simulink model "s_heli3d_cnn"  (R2023a)
settings: Solver=ode1  StartTime=0.0  StopTime=30  FixedStep=0.002  RelTol=1e-3  EnableMultiTasking=on
model workspace (MAT data in the model file):
  helicopter_models.Mdl = SeriesNetwork
  helicopter_models.Mdl.any.Version = 1
  helicopter_models.Mdl.any.Layers(1) = nnet.cnn.layer.FeatureInputLayer
  helicopter_models.Mdl.any.Layers(1).any.Version = 2
  helicopter_models.Mdl.any.Layers(1).any.Name = 'input'
  helicopter_models.Mdl.any.Layers(1).any.InputSize = 9
  helicopter_models.Mdl.any.Layers(1).any.Normalization = []
  helicopter_models.Mdl.any.Layers(1).any.NormalizationDimension = 'auto'
  helicopter_models.Mdl.any.Layers(1).any.SplitComplexInputs = 0
  helicopter_models.Mdl.any.Layers(2) = nnet.cnn.layer.FullyConnectedLayer
  helicopter_models.Mdl.any.Layers(2).any.Version = 3
  helicopter_models.Mdl.any.Layers(2).any.Name = 'fc1'
  helicopter_models.Mdl.any.Layers(2).any.InputSize = 9
  helicopter_models.Mdl.any.Layers(2).any.OutputSize = 256
  helicopter_models.Mdl.any.Layers(2).any.Weights.Version = 2
  helicopter_models.Mdl.any.Layers(2).any.Weights.Value = [0.13310675323 0.208178877831 -0.160442724824 0.136672541499 0.137998655438 0.0987144708633 0.0352399460971 -0.192555785179 0.245779588819 0.00993849057704 -0.0564966723323 -0.160766735673 ... (2304 elements, 256x9)]
  helicopter_models.Mdl.any.Layers(2).any.Weights.LearnRateFactor = 1
  helicopter_models.Mdl.any.Layers(2).any.Weights.L2Factor = 1
  helicopter_models.Mdl.any.Layers(2).any.Weights.Initializer.Version = 1
  helicopter_models.Mdl.any.Layers(2).any.Weights.Initializer.Class = 'nnet.internal.cnn.layer.learnable.initializer.Glorot'
  helicopter_models.Mdl.any.Layers(2).any.Weights.Initializer.ConstructorArguments = {2, 1}
  helicopter_models.Mdl.any.Layers(2).any.Bias.Version = 2
  helicopter_models.Mdl.any.Layers(2).any.Bias.Value = [0.149443045259 0.102787695825 0.0137507077307 -0.0149580715224 -0.377757281065 0.0530572384596 -0.0382270552218 0.0523963347077 0.0614480637014 -0.112386830151 -0.0184559673071 0.0208104513586 ... (256 elements, 256x1)]
  helicopter_models.Mdl.any.Layers(2).any.Bias.LearnRateFactor = 1
  helicopter_models.Mdl.any.Layers(2).any.Bias.L2Factor = 0
  helicopter_models.Mdl.any.Layers(2).any.Bias.Initializer.Version = 1
  helicopter_models.Mdl.any.Layers(2).any.Bias.Initializer.Class = 'nnet.internal.cnn.layer.learnable.initializer.Zeros'
  helicopter_models.Mdl.any.Layers(2).any.Bias.Initializer.ConstructorArguments = []
  helicopter_models.Mdl.any.Layers(3) = nnet.cnn.layer.TanhLayer
  helicopter_models.Mdl.any.Layers(3).Name = 'tanh1'
  helicopter_models.Mdl.any.Layers(3).Description = 'Hyperbolic tangent'
  helicopter_models.Mdl.any.Layers(3).Type = 'Tanh'
  helicopter_models.Mdl.any.Layers(3).PrivateNumStates = 0
  helicopter_models.Mdl.any.Layers(4) = nnet.cnn.layer.FullyConnectedLayer
  helicopter_models.Mdl.any.Layers(4).any.Version = 3
  helicopter_models.Mdl.any.Layers(4).any.Name = 'fc2'
  helicopter_models.Mdl.any.Layers(4).any.InputSize = 256
  helicopter_models.Mdl.any.Layers(4).any.OutputSize = 256
  helicopter_models.Mdl.any.Layers(4).any.Weights.Version = 2
  helicopter_models.Mdl.any.Layers(4).any.Weights.Value = [0.0176317542791 -0.0498906224966 -0.00331918848678 -0.0305134225637 -0.000809711986221 0.0326992608607 0.0677321329713 -0.0315245091915 0.0983166620135 0.00188921799418 -0.136850476265 -0.0060957390815 ... (65536 elements, 256x256)]
  helicopter_models.Mdl.any.Layers(4).any.Weights.LearnRateFactor = 1
  helicopter_models.Mdl.any.Layers(4).any.Weights.L2Factor = 1
  helicopter_models.Mdl.any.Layers(4).any.Weights.Initializer.Version = 1
  helicopter_models.Mdl.any.Layers(4).any.Weights.Initializer.Class = 'nnet.internal.cnn.layer.learnable.initializer.Glorot'
  helicopter_models.Mdl.any.Layers(4).any.Weights.Initializer.ConstructorArguments = {2, 1}
  helicopter_models.Mdl.any.Layers(4).any.Bias.Version = 2
  helicopter_models.Mdl.any.Layers(4).any.Bias.Value = [-0.000405726634199 -0.174336075783 -0.000397357915062 0.0493232049048 -0.0152544146404 0.137321993709 0.0236514117569 0.0224169250578 0.156086027622 -0.0284760966897 -0.181728631258 0.00929012987763 ... (256 elements, 256x1)]
  helicopter_models.Mdl.any.Layers(4).any.Bias.LearnRateFactor = 1
  helicopter_models.Mdl.any.Layers(4).any.Bias.L2Factor = 0
  helicopter_models.Mdl.any.Layers(4).any.Bias.Initializer.Version = 1
  helicopter_models.Mdl.any.Layers(4).any.Bias.Initializer.Class = 'nnet.internal.cnn.layer.learnable.initializer.Zeros'
  helicopter_models.Mdl.any.Layers(4).any.Bias.Initializer.ConstructorArguments = []
  helicopter_models.Mdl.any.Layers(5) = nnet.cnn.layer.TanhLayer
  helicopter_models.Mdl.any.Layers(5).Name = 'tanh2'
  helicopter_models.Mdl.any.Layers(5).Description = 'Hyperbolic tangent'
  helicopter_models.Mdl.any.Layers(5).Type = 'Tanh'
  helicopter_models.Mdl.any.Layers(5).PrivateNumStates = 0
  helicopter_models.Mdl.any.Layers(6) = nnet.cnn.layer.FullyConnectedLayer
  helicopter_models.Mdl.any.Layers(6).any.Version = 3
  helicopter_models.Mdl.any.Layers(6).any.Name = 'fc3'
  helicopter_models.Mdl.any.Layers(6).any.InputSize = 256
  helicopter_models.Mdl.any.Layers(6).any.OutputSize = 64
  helicopter_models.Mdl.any.Layers(6).any.Weights.Version = 2
  helicopter_models.Mdl.any.Layers(6).any.Weights.Value = [-0.0452437326312 0.0290121845901 -0.0681063830853 0.0147047163919 0.0793885588646 0.0247011203319 -0.0402223840356 0.00778562109917 -0.00158385897521 -0.0439031943679 0.0822357684374 0.0465763583779 ... (16384 elements, 64x256)]
  helicopter_models.Mdl.any.Layers(6).any.Weights.LearnRateFactor = 1
  helicopter_models.Mdl.any.Layers(6).any.Weights.L2Factor = 1
  helicopter_models.Mdl.any.Layers(6).any.Weights.Initializer.Version = 1
  helicopter_models.Mdl.any.Layers(6).any.Weights.Initializer.Class = 'nnet.internal.cnn.layer.learnable.initializer.Glorot'
  helicopter_models.Mdl.any.Layers(6).any.Weights.Initializer.ConstructorArguments = {2, 1}
  helicopter_models.Mdl.any.Layers(6).any.Bias.Version = 2
  helicopter_models.Mdl.any.Layers(6).any.Bias.Value = [-0.0450097173452; 0.110222563148; 0.0499272234738; -0.256927847862; -0.0182336308062; 0.0690494850278; -0.0224842149764; -0.0260149128735; -0.0677949637175; 0.0852068662643; 0.0772904083133; -0.041886292398; -0.0397085435688; 0.0259099658579; 0.196818158031; -0.0621182322502; 0.0445226170123; -0.126585230231; -0.107752278447; 0.0519631318748; -0.000391898822272; 0.0276712477207; -0.0782154947519; 0.032532338053; -0.0242742709816; -0.0756259560585; 0.0465251728892; 0.0445563457906; -0.104431308806; -0.0272272955626; -0.0313442610204; -0.106223650277; 0.00512412656099; 0.0870658904314; -0.0178943593055; -0.0364487729967; -0.0710658580065; -0.118151128292; 0.0517238453031; -0.0601879768074; -0.082881256938; 0.0530342683196; 0.0417108535767; -0.0169844310731; -0.057533249259; -0.0626719966531; -0.0924978479743; 0.106941841543; 0.0436584912241; 0.0255041811615; -0.035246014595; -0.0307711735368; -0.12418603152; 0.0192781593651; -0.0865231901407; 0.232267320156; 0.00646506296471; 0.0691988766193; 0.0548212714493; -0.0892309471965; -0.039018008858; 0.146687179804; -0.0416509397328; 0.0172210410237]
  helicopter_models.Mdl.any.Layers(6).any.Bias.LearnRateFactor = 1
  helicopter_models.Mdl.any.Layers(6).any.Bias.L2Factor = 0
  helicopter_models.Mdl.any.Layers(6).any.Bias.Initializer.Version = 1
  helicopter_models.Mdl.any.Layers(6).any.Bias.Initializer.Class = 'nnet.internal.cnn.layer.learnable.initializer.Zeros'
  helicopter_models.Mdl.any.Layers(6).any.Bias.Initializer.ConstructorArguments = []
  helicopter_models.Mdl.any.Layers(7) = nnet.cnn.layer.TanhLayer
  helicopter_models.Mdl.any.Layers(7).Name = 'tanh3'
  helicopter_models.Mdl.any.Layers(7).Description = 'Hyperbolic tangent'
  helicopter_models.Mdl.any.Layers(7).Type = 'Tanh'
  helicopter_models.Mdl.any.Layers(7).PrivateNumStates = 0
  helicopter_models.Mdl.any.Layers(8) = nnet.cnn.layer.FullyConnectedLayer
  helicopter_models.Mdl.any.Layers(8).any.Version = 3
  helicopter_models.Mdl.any.Layers(8).any.Name = 'fc_out'
  helicopter_models.Mdl.any.Layers(8).any.InputSize = 64
  helicopter_models.Mdl.any.Layers(8).any.OutputSize = 2
  helicopter_models.Mdl.any.Layers(8).any.Weights.Version = 2
  helicopter_models.Mdl.any.Layers(8).any.Weights.Value = [0.399694085121 0.323152422905 -0.531250953674 -0.462554991245 0.173690021038 -0.378186702728 0.179041266441 0.223057076335 0.29842659831 0.168712005019 -0.037637218833 0.235301449895 ... (128 elements, 2x64)]
  helicopter_models.Mdl.any.Layers(8).any.Weights.LearnRateFactor = 1
  helicopter_models.Mdl.any.Layers(8).any.Weights.L2Factor = 1
  helicopter_models.Mdl.any.Layers(8).any.Weights.Initializer.Version = 1
  helicopter_models.Mdl.any.Layers(8).any.Weights.Initializer.Class = 'nnet.internal.cnn.layer.learnable.initializer.Glorot'
  helicopter_models.Mdl.any.Layers(8).any.Weights.Initializer.ConstructorArguments = {2, 1}
  helicopter_models.Mdl.any.Layers(8).any.Bias.Version = 2
  helicopter_models.Mdl.any.Layers(8).any.Bias.Value = [-0.0146038485691; -0.0499037839472]
  helicopter_models.Mdl.any.Layers(8).any.Bias.LearnRateFactor = 1
  helicopter_models.Mdl.any.Layers(8).any.Bias.L2Factor = 0
  helicopter_models.Mdl.any.Layers(8).any.Bias.Initializer.Version = 1
  helicopter_models.Mdl.any.Layers(8).any.Bias.Initializer.Class = 'nnet.internal.cnn.layer.learnable.initializer.Zeros'
  helicopter_models.Mdl.any.Layers(8).any.Bias.Initializer.ConstructorArguments = []
  helicopter_models.Mdl.any.Layers(9) = nnet.cnn.layer.RegressionOutputLayer
  helicopter_models.Mdl.any.Layers(9).any.Version = 2
  helicopter_models.Mdl.any.Layers(9).any.Name = 'reg'
  helicopter_models.Mdl.any.Layers(9).any.ResponseNames = {'Response'}
  helicopter_models.Mdl.any.Layers(9).any.ObservationDim = 2
  helicopter_models.muX = [0.00841649414055 0.000984354131905 0.0278180475455 -0.00241604057039 -0.00234545060113 -0.00253481813169 0.020325458386 0.00106425674144 0.0323945886649]
  helicopter_models.sigX = [0.195795117535 0.11238391609 0.233261557044 0.202451978779 0.279333503069 0.0990159398718 0.248410084503 0.123809358025 0.225516865567]
  helicopter_models.muY = [0.0199933353292 0.0223974644218]
  helicopter_models.sigY = [2.61588215573 2.71489296905]
  helicopter_models.K = [51.9211238898  27.977022009  -16.7090306849  24.6003547305  6.93916669558  -27.9984963147  14.1421356237  -1.41421356237; 51.9211238898  -27.977022009  16.7090306849  24.6003547305  -6.93916669558  27.9984963147  14.1421356237  1.41421356237]
values from neighbouring files (symbols this model uses):
  A = sys.A    [read_model.m]
  B = sys.B    [read_model.m]
  CMD_RATE_LIMIT = 45.0 * pi / 180    (= 0.785398163397)    [setup_lab_heli_3d.m]
  D = zeros(6,2)    [trained.m]
  K_AMP = 3    [setup_lab_heli_3d.m]
  muX = helicopter_models.muX    [read_model.m]    (also in trained.m = mean(X,1))
  muY = helicopter_models.muY    [read_model.m]    (also in trained.m = mean(Y,1))
  sigX = helicopter_models.sigX    [read_model.m]    (also in trained.m = std(X,[],1) + 1e-9)
  sigY = helicopter_models.sigY    [read_model.m]    (also in trained.m = std(Y,[],1) + 1e-9)
  VMAX_AMP = 24    [setup_lab_heli_3d.m]
  VMAX_DAC = 10    [setup_lab_heli_3d.m]
libraries: simulink_extras x3, deeplib x1
settings Model: ExtModeTrigDuration=5000  Creator=MLevis  LastModifiedBy=hackbrian
settings SolverCC: AlgebraicLoopSolver=TrustRegion  PositivePriorityOrder=on
settings DataIOCC: LimitDataPoints=on  SaveFormat=Array  SignalLoggingSaveFormat=ModelDataLogs  ReturnWorkspaceOutputs=off
settings OptimizationCC: BooleanDataType=off  OptimizeBlockIOStorage=off  BufferReuse=off  ExpressionFolding=off  ExpressionDepthLimit=2147483647  LocalBlockOutputs=off  InitFltsAndDblsToZero=on
settings DebuggingCC: SaveWithParameterizedLinksMsg=none  UnderspecifiedInitializationDetection=Classic  MergeDetectMultiDrivingBlocksExec=none  SignalResolutionControl=TryResolveAllWithWarning  SolverPrmCheckMsg=warning  MultiTaskDSMMsg=warning  MultiTaskCondExecSysMsg=none  FcnCallInpInsideContextMsg=warning  UnconnectedInputMsg=warning  UnconnectedOutputMsg=warning  UnconnectedLineMsg=warning  StateNameClashWarn=warning  SFUnexpectedBacktrackingDiag=warning  SFNoUnconditionalDefaultTransitionDiag=warning  SFExecutionAtInitializationDiag=none  ArithmeticOperatorsInVariantConditions=warning
settings ModelReferenceCC: PropagateSignalLabelsOutOfModel=off
settings SFSimCC: SimTargetLang=C++
settings CodeAppCC: StateflowObjectComments=on
settings GRTTargetCC: TargetLangStandard=C89/C90 (ANSI)
settings ConfigComp: CovMetricSettings=dw  CovSaveCumulativeToWorkspaceVar=on  CovSaveSingleToWorkspaceVar=on

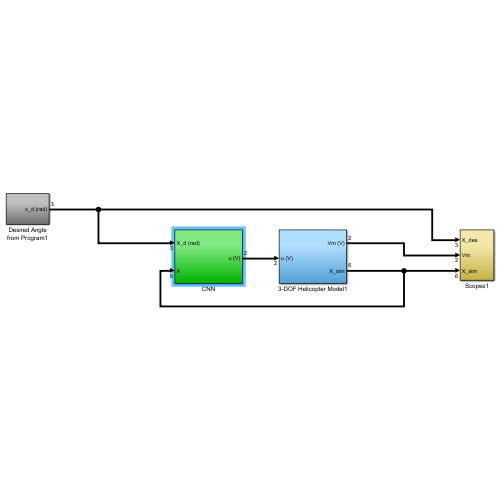
[thumbnail: Simulink's stored preview of the top-level diagram]
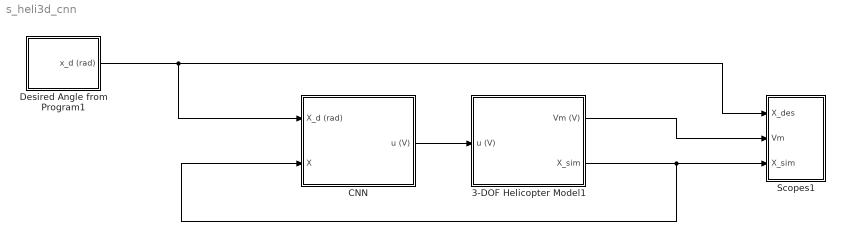
== system s_heli3d_cnn ==
  3-DOF Helicopter Model1 : Subsystem
  CNN : Subsystem  AncestorBlock=heli_2d_lib/2DOF HELI: FF+LQR+I Controller
      settings: LibrarySourceBlock=|
      | heli_2d_lib/2DOF HELI:
      | FF+LQR+I Controller
  Desired Angle from Program1 : Subsystem
  Scopes1 : Subsystem
  wires:
  3-DOF Helicopter Model1/2(X_sim) -> CNN/2(X), Scopes1/3(X_sim)
  Desired Angle from Program1/1(x_d (rad)) -> CNN/1(X_d (rad)), Scopes1/1(X_des)
  3-DOF Helicopter Model1/1(Vm (V)) -> Scopes1/2(Vm)
  CNN/1(u (V)) -> 3-DOF Helicopter Model1/1(u (V))

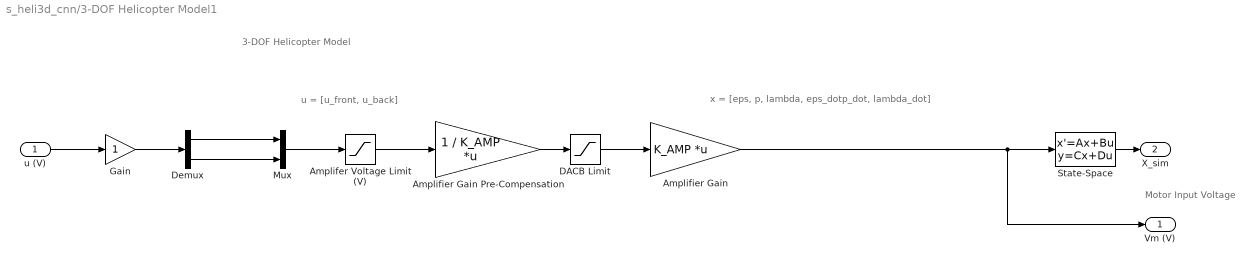
== system s_heli3d_cnn/3-DOF Helicopter Model1 ==
  note: x = [eps, p, lambda, eps_dotp_dot, lambda_dot]
  note: u = [u_front, u_back]
  note: Motor Input Voltage
  note: 3-DOF Helicopter Model
  u (V) : Inport
  Amplifer Voltage Limit (V) : Saturate  UpperLimit=VMAX_AMP  LowerLimit=-VMAX_AMP
  Amplifier Gain : Gain  Gain=K_AMP  Multiplication=Matrix(K*u)  SaturateOnIntegerOverflow=on  OutDataTypeStr=Inherit: Same as input  ParamDataTypeStr=Inherit: Same as input
  Amplifier Gain Pre-Compensation : Gain  Gain=1 / K_AMP  Multiplication=Matrix(K*u)  SaturateOnIntegerOverflow=on  OutDataTypeStr=Inherit: Same as input  ParamDataTypeStr=Inherit: Same as input
  DACB Limit : Saturate  UpperLimit=VMAX_DAC  LowerLimit=-VMAX_DAC
  Demux : Demux  Outputs=2
  Gain : Gain
  Mux : Mux  Inputs=2
  State-Space : StateSpace  A=A  B=B  C=eye(6,6)  D=zeros(6,2)  InitialCondition=0
  Vm (V) : Outport
  X_sim : Outport  Port=2
  wires:
  State-Space/1 -> X_sim/1
  Amplifer Voltage Limit (V)/1 -> Amplifier Gain Pre-Compensation/1
  Amplifier Gain Pre-Compensation/1 -> DACB Limit/1
  DACB Limit/1 -> Amplifier Gain/1
  Amplifier Gain/1 -> Vm (V)/1, State-Space/1
  Mux/1 -> Amplifer Voltage Limit (V)/1
  u (V)/1 -> Gain/1
  Demux/2 -> Mux/2
  Demux/1 -> Mux/1
  Gain/1 -> Demux/1

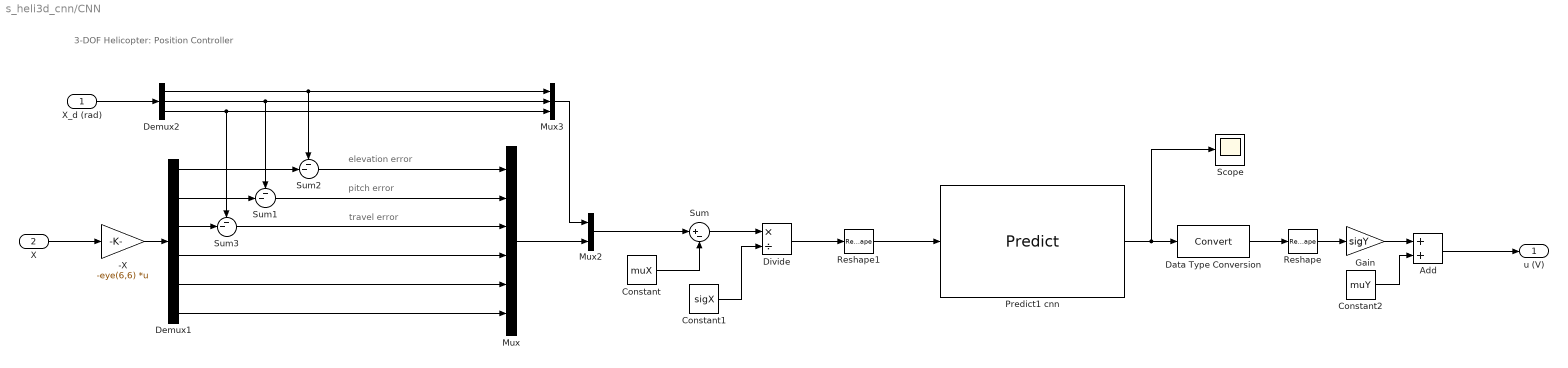
== system s_heli3d_cnn/CNN ==
  note: elevation error
  note: pitch error
  note: 3-DOF Helicopter: Position Controller
  note: travel error
  X_d (rad) : Inport
  X : Inport  Port=2
  -X : Gain  Gain=-eye(6,6)  Multiplication=Matrix(K*u)
  Add : Sum
  Constant : Constant  Value=muX
  Constant1 : Constant  Value=sigX
  Constant2 : Constant  Value=muY
  Data Type Conversion : DataTypeConversion  SaturateOnIntegerOverflow=off  RndMeth=Floor
  Demux1 : Demux  Outputs=6
  Demux2 : Demux  Outputs=3
  Divide : Product  Inputs=*/
  Gain : Gain  Gain=sigY
  Mux : Mux  Inputs=6
  Mux2 : Mux  Inputs=2
  Mux3 : Mux  Inputs=3
  Predict1 cnn : deeplib/Predict  Network=Network from MAT-file  NetworkFunction=squeezenet  NetworkFilePath=/home/hackbrian/Documents/Courseware Resources_Heli/Advanced Applications/CNN/Model_helicopter_direct_controller.mat  MiniBatchSize=128  InputDataFormats={'',''}  Predictions=on  Activations={}  ForceInterpretedSim=off  EnableDLNetwork=on
  Reshape : Reshape  OutputDimensionality=Customize  OutputDimensions=[2]
  Reshape1 : Reshape  OutputDimensionality=Row vector (2-D)
  Scope : Scope
  Sum : Sum  Inputs=|+-
  Sum1 : Sum  Inputs=--|
  Sum2 : Sum  Inputs=--|
  Sum3 : Sum  Inputs=--|
  u (V) : Outport
  wires:
  Demux1/2 -> Sum1/2
  Demux2/2 -> Mux3/2, Sum1/1
  Demux2/1 -> Mux3/1, Sum2/1
  X_d (rad)/1 -> Demux2/1
  Demux1/1 -> Sum2/2
  X/1 -> -X/1
  Sum1/1 -> Mux/2
  -X/1 -> Demux1/1
  Demux2/3 -> Sum3/1, Mux3/3
  Demux1/3 -> Sum3/2
  Sum3/1 -> Mux/3
  Demux1/4 -> Mux/4
  Demux1/5 -> Mux/5
  Demux1/6 -> Mux/6
  Sum2/1 -> Mux/1
  Reshape1/1 -> Predict1 cnn/1
  Mux/1 -> Mux2/2
  Reshape/1 -> Gain/1
  Data Type Conversion/1 -> Reshape/1
  Mux2/1 -> Sum/1
  Mux3/1 -> Mux2/1
  Constant/1 -> Sum/2
  Sum/1 -> Divide/1
  Constant1/1 -> Divide/2
  Divide/1 -> Reshape1/1
  Add/1 -> u (V)/1
  Gain/1 -> Add/1
  Constant2/1 -> Add/2
  Predict1 cnn/1 -> Scope/1, Data Type Conversion/1

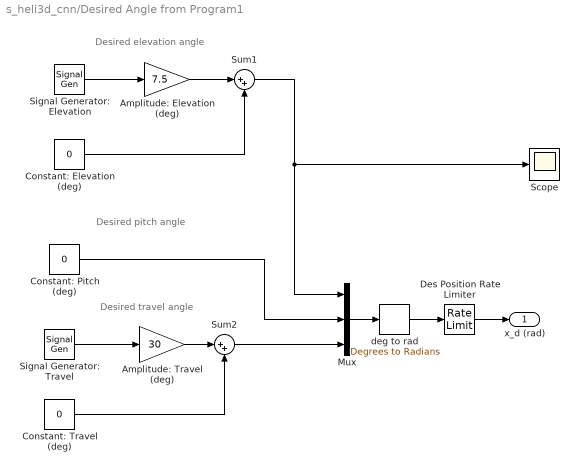
== system s_heli3d_cnn/Desired Angle from Program1 ==
  note: Desired elevation angle
  note: Desired travel angle
  note: Desired pitch angle
  Amplitude: Elevation (deg) : Gain  Gain=7.5
  Amplitude: Travel (deg) : Gain  Gain=30
  Constant: Elevation (deg) : Constant  Value=0
  Constant: Pitch (deg) : Constant  Value=0
  Constant: Travel (deg) : Constant  Value=0
  Des Position Rate Limiter : RateLimiter  RisingSlewLimit=CMD_RATE_LIMIT  FallingSlewLimit=-CMD_RATE_LIMIT  SampleTimeMode=inherited
  Mux : Mux  Inputs=3
  Scope : Scope
  Signal Generator: Elevation : SignalGenerator  WaveForm=square  Frequency=0.04
  Signal Generator: Travel : SignalGenerator  WaveForm=square  Frequency=0.03
  Sum1 : Sum  Inputs=|++
  Sum2 : Sum  Inputs=|++
  deg to rad : simulink_extras/Transformations/Degrees to Radians
  x_d (rad) : Outport
  wires:
  Mux/1 -> deg to rad/1
  Constant: Elevation (deg)/1 -> Sum1/2
  Amplitude: Elevation (deg)/1 -> Sum1/1
  Signal Generator: Elevation/1 -> Amplitude: Elevation (deg)/1
  Constant: Travel (deg)/1 -> Sum2/2
  Signal Generator: Travel/1 -> Amplitude: Travel (deg)/1
  deg to rad/1 -> Des Position Rate Limiter/1
  Constant: Pitch (deg)/1 -> Mux/2
  Sum1/1 -> Mux/1, Scope/1
  Des Position Rate Limiter/1 -> x_d (rad)/1
  Amplitude: Travel (deg)/1 -> Sum2/1
  Sum2/1 -> Mux/3

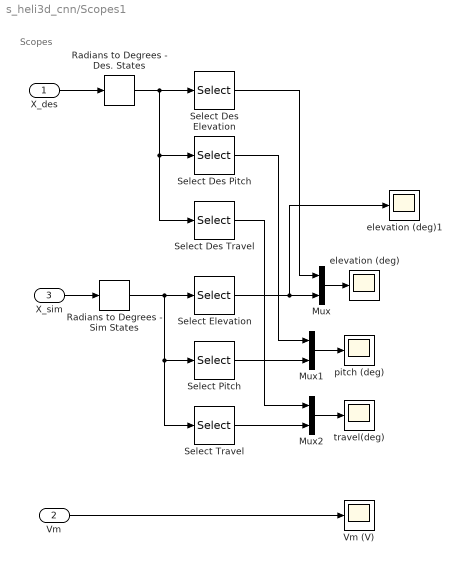
== system s_heli3d_cnn/Scopes1 ==
  note: Scopes
  X_des : Inport
  Vm : Inport  Port=2
  X_sim : Inport  Port=3
  Mux : Mux  Inputs=2
  Mux1 : Mux  Inputs=2
  Mux2 : Mux  Inputs=2
  Radians to Degrees - Des. States : simulink_extras/Transformations/Radians to Degrees
  Radians to Degrees - Sim States : simulink_extras/Transformations/Radians to Degrees
  Select Des Elevation : Selector  InputPortWidth=3  IndexOptions=Index vector (dialog)  Indices=1  OutputSizes=1
  Select Des Pitch : Selector  InputPortWidth=3  IndexOptions=Index vector (dialog)  Indices=2  OutputSizes=1
  Select Des Travel : Selector  InputPortWidth=3  IndexOptions=Index vector (dialog)  Indices=3  OutputSizes=1
  Select Elevation : Selector  InputPortWidth=6  IndexOptions=Index vector (dialog)  Indices=1  OutputSizes=1
  Select Pitch : Selector  InputPortWidth=6  IndexOptions=Index vector (dialog)  Indices=2  OutputSizes=1
  Select Travel : Selector  InputPortWidth=6  IndexOptions=Index vector (dialog)  Indices=3  OutputSizes=1
  Vm (V) : Scope
  elevation (deg) : Scope
  elevation (deg)1 : Scope
  pitch (deg) : Scope
  travel(deg) : Scope
  wires:
  X_des/1 -> Radians to Degrees - Des. States/1
  X_sim/1 -> Radians to Degrees - Sim States/1
  Mux/1 -> elevation (deg)/1
  Mux1/1 -> pitch (deg)/1
  Vm/1 -> Vm (V)/1
  Radians to Degrees - Sim States/1 -> Select Elevation/1, Select Pitch/1, Select Travel/1
  Mux2/1 -> travel(deg)/1
  Select Elevation/1 -> Mux/2, elevation (deg)1/1
  Select Pitch/1 -> Mux1/2
  Select Travel/1 -> Mux2/2
  Radians to Degrees - Des. States/1 -> Select Des Elevation/1, Select Des Pitch/1, Select Des Travel/1
  Select Des Elevation/1 -> Mux/1
  Select Des Pitch/1 -> Mux1/1
  Select Des Travel/1 -> Mux2/1
